simulink model "rct_airframeGS"  (R2016b)
settings: Solver=ode45  StartTime=0.0  StopTime=50  RelTol=1e-3  AbsTol=1e-6
PreLoadFcn:
  | x_ini = 0;
  | h_ini = 10000/3.28084;  % 10,000 ft
  | alpha_ini = 0;
  | theta_ini = 0;
  | v_ini = 700;   % m/s
  | q_ini = 0;
model workspace (MATLAB code in the model file):
  | AirframeData
  | Kp0 = 0.1*ones(11,8);
  | Ki0 = 2*ones(11,8);
  | Ka0 = 0.001*ones(11,8);
  | Kg0 = -1000*ones(11,8);
undefined symbols (not defined in the file or in its folder): Cm_alpha, Cm_el, Cm_q, Cx_alpha, Cz_alpha, Cz_el, d2r, d_ref, fin_max, fin_min, g, S_ref, Thrust
libraries: aerospace x3, simulink x1
settings Model: ExtModeTrigMode=oneshot  ExtModeArmWhenConnect=off  ExtModeAutoUpdateStatusClock=off  Creator=The MathWorks, Inc.  LastModifiedBy=The MathWorks, Inc.
settings DataIOCC: SaveFormat=Array  SignalLoggingName=sigsOut
settings OptimizationCC: BlockReduction=off  BooleanDataType=off  ExpressionDepthLimit=2147483647  InitFltsAndDblsToZero=on  LifeSpan=inf
settings DebuggingCC: SaveWithParameterizedLinksMsg=none  UnderspecifiedInitializationDetection=Classic  MergeDetectMultiDrivingBlocksExec=none  CheckExecutionContextPreStartOutputMsg=on  CheckExecutionContextRuntimeOutputMsg=on  SignalResolutionControl=TryResolveAllWithWarning  MultiTaskDSMMsg=warning  FcnCallInpInsideContextMsg=warning  AllowSymbolicDim=off  StateNameClashWarn=warning  SFUnexpectedBacktrackingDiag=warning  SFNoUnconditionalDefaultTransitionDiag=warning  SFExecutionAtInitializationDiag=none
settings HardwareCC: ProdBitPerPointer=32  ProdBitPerSizeT=32  ProdBitPerPtrDiffT=32  ProdLargestAtomicFloat=None  ProdIntDivRoundTo=Undefined  ProdEndianess=Unspecified  ProdWordSize=32  ProdHWDeviceType=32-bit Generic  TargetUnknown=on
settings ModelReferenceCC: PropagateSignalLabelsOutOfModel=off
settings GRTTargetCC: TargetFcnLib=ansi_tfl_tmw.mat  TargetLangStandard=C89/C90 (ANSI)  GeneratePreprocessorConditionals=Disable all  CombineOutputUpdateFcns=off  GRTInterface=on
settings ConfigComp: CovMetricSettings=dw  CovHtmlReporting=on  CovSaveCumulativeToWorkspaceVar=on  CovSaveSingleToWorkspaceVar=on  CovExternalEMLEnable=off

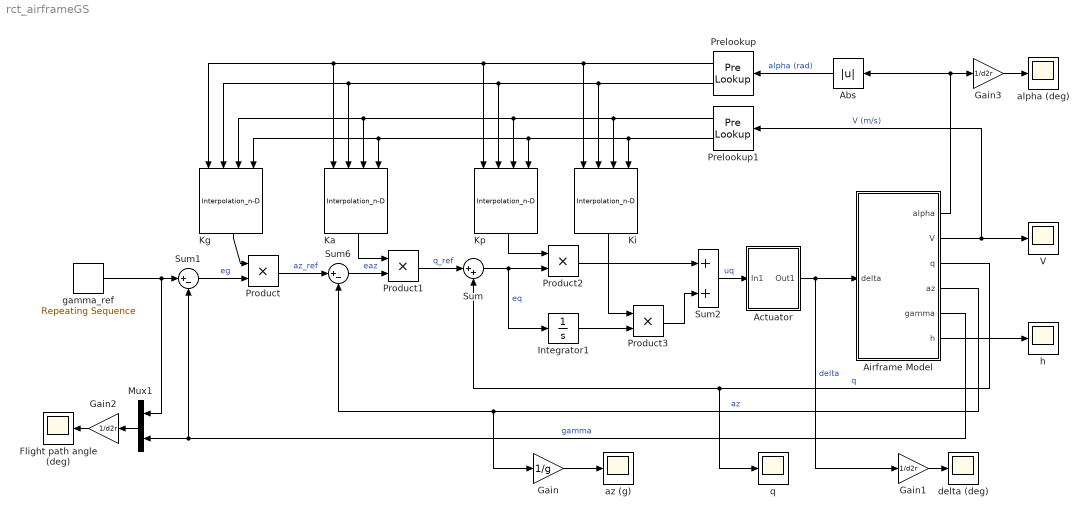
== system rct_airframeGS ==
  Abs : Abs
  Actuator : Subsystem
  Airframe Model : Subsystem
  Flight path angle (deg) : Scope
  Gain : Gain  Gain=1/g
  Gain1 : Gain  Gain=1/d2r
  Gain2 : Gain  Gain=1/d2r
  Gain3 : Gain  Gain=1/d2r
  Integrator1 : Integrator
  Ka : Interpolation_n-D  Table=Ka0  InternalRulePriority=Speed
  Kg : Interpolation_n-D  Table=Kg0  InternalRulePriority=Speed
  Ki : Interpolation_n-D  Table=Ki0  InternalRulePriority=Speed
  Kp : Interpolation_n-D  Table=Kp0  InternalRulePriority=Speed
  Mux1 : Mux  Inputs=2
  Prelookup : PreLookup  BreakpointsData=(0:2:20)*(pi/180)  ExtrapMethod=Linear
  Prelookup1 : PreLookup  BreakpointsData=700:100:1400  ExtrapMethod=Linear
  Product{,1..3} (4 alike) : Product
  Sum : Sum  Inputs=|++  SaturateOnIntegerOverflow=on
  Sum1 : Sum  Inputs=|+-  SaturateOnIntegerOverflow=on
  Sum2 : Sum  SaturateOnIntegerOverflow=on
  Sum6 : Sum  Inputs=|+-  SaturateOnIntegerOverflow=on
  V : Scope
  alpha (deg) : Scope
  az (g) : Scope
  delta (deg) : Scope
  gamma_ref : simulink/Sources/Repeating Sequence  rep_seq_t=[0 6 8 16 20 26 32 40 44 50]  rep_seq_y=[0 0 pi/6 pi/6 -pi/6 -pi/6 pi/4 pi/4 0 0]
  h : Scope
  q : Scope
  wires:
  Sum/1 -> Product2/2, Integrator1/1  "eq"
  Product3/1 -> Sum2/2
  Airframe Model/4(az) -> Gain/1, Sum6/2  "az"
  Airframe Model/1(alpha) -> Abs/1, Gain3/1
  Product2/1 -> Sum2/1
  Product1/1 -> Sum/1  "q_ref"
  Sum6/1 -> Product1/2  "eaz"
  Actuator/1(Out1) -> Airframe Model/1(delta), Gain1/1  "delta"
  Product/1 -> Sum6/1  "az_ref"
  Sum1/1 -> Product/2  "eg"
  Airframe Model/5(gamma) -> Mux1/2, Sum1/2  "gamma"
  Sum2/1 -> Actuator/1(In1)  "uq"
  Airframe Model/3(q) -> q/1, Sum/2  "q"
  gamma_ref/1 -> Sum1/1, Mux1/1
  Gain/1 -> az (g)/1
  Gain1/1 -> delta (deg)/1
  Mux1/1 -> Gain2/1
  Gain2/1 -> Flight path angle (deg)/1
  Gain3/1 -> alpha (deg)/1
  Airframe Model/2(V) -> Prelookup1/1, V/1  "V (m/s)"
  Airframe Model/6(h) -> h/1
  Kg/1 -> Product/1
  Ka/1 -> Product1/1
  Integrator1/1 -> Product3/2
  Kp/1 -> Product2/1
  Ki/1 -> Product3/1
  Abs/1 -> Prelookup/1  "alpha (rad)"
  Prelookup/1 -> Ka/1, Kg/1, Kp/1, Ki/1
  Prelookup/2 -> Ki/2, Kp/2, Ka/2, Kg/2
  Prelookup1/1 -> Kp/3, Kg/3, Ka/3, Ki/3
  Prelookup1/2 -> Ki/4, Kg/4, Ka/4, Kp/4

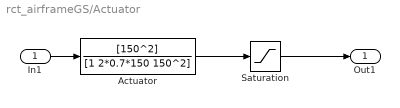
== system rct_airframeGS/Actuator ==
  In1 : Inport
  Actuator : TransferFcn  Numerator=[150^2]  Denominator=[1 2*0.7*150 150^2]
  Saturation : Saturate  UpperLimit=fin_max  LowerLimit=fin_min
  Out1 : Outport
  wires:
  Actuator/1 -> Saturation/1
  In1/1 -> Actuator/1
  Saturation/1 -> Out1/1

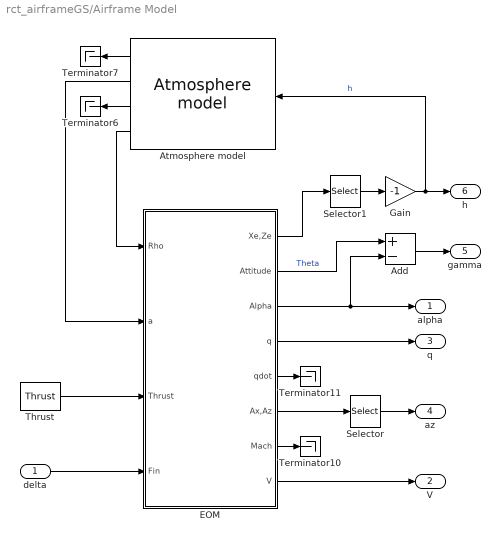
== system rct_airframeGS/Airframe Model ==
  delta : Inport
  Add : Sum  Inputs=+-
  Atmosphere model : aerospace/Atmosphere/Atmosphere model
  EOM : Subsystem
  Gain : Gain  Gain=-1
  Selector : Selector  InputPortWidth=2  IndexOptions=Index vector (dialog)  Indices=[2]  OutputSizes=1
  Selector1 : Selector  InputPortWidth=2  IndexOptions=Index vector (dialog)  Indices=[2]  OutputSizes=1
  Terminator{6..7,10..11} (4 alike) : Terminator
  Thrust : Constant  Value=Thrust
  alpha : Outport  InitialOutput=0
  V : Outport  Port=2  InitialOutput=0
  q : Outport  Port=3  InitialOutput=0
  az : Outport  Port=4  InitialOutput=0
  gamma : Outport  Port=5  InitialOutput=0
  h : Outport  Port=6  InitialOutput=0
  wires:
  Atmosphere model/1 -> Terminator7/1
  Atmosphere model/3 -> Terminator6/1
  delta/1 -> EOM/4(Fin)
  EOM/8(V) -> V/1
  Selector/1 -> az/1
  Atmosphere model/2 -> EOM/2(a)
  Atmosphere model/4 -> EOM/1(Rho)
  EOM/7(Mach) -> Terminator10/1
  EOM/5(qdot) -> Terminator11/1
  EOM/4(q) -> q/1
  Thrust/1 -> EOM/3(Thrust)
  EOM/3(Alpha) -> alpha/1, Add/2
  EOM/6(Ax,Az) -> Selector/1
  EOM/2(Attitude) -> Add/1  "Theta"
  Add/1 -> gamma/1
  EOM/1(Xe,Ze) -> Selector1/1
  Selector1/1 -> Gain/1
  Gain/1 -> Atmosphere model/1, h/1  "h"

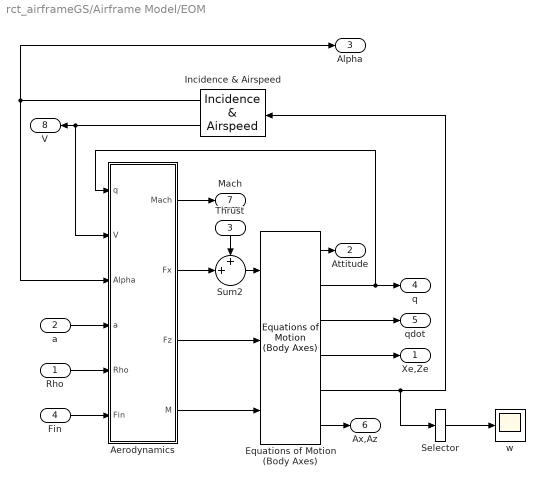
== system rct_airframeGS/Airframe Model/EOM ==
  Rho : Inport
  a : Inport  Port=2
  Thrust : Inport  Port=3
  Fin : Inport  Port=4
  " Equations of Motion (Body Axes)" : aerospace/3DoF Equations of Motion / Equations of Motion (Body Axes)  v_ini=v_ini  theta_ini=theta_ini  alpha_ini=alpha_ini  q_ini=q_ini  pos_ini=[x_ini -h_ini]  mass=mass  Iyy=Iyy  g=g
  Aerodynamics : Subsystem
  Incidence & Airspeed : aerospace/3DoF Equations of Motion /Incidence  & Airspeed
  Selector : Selector  InputPortWidth=2  IndexOptions=Index vector (dialog)  Indices=[2]  OutputSizes=1
  Sum2 : Sum  Inputs=++|  SaturateOnIntegerOverflow=on  InputSameDT=on  OutDataTypeStr=Inherit: Same as first input
  w : Scope
  Xe,Ze : Outport  InitialOutput=0
  Attitude : Outport  Port=2  InitialOutput=0
  Alpha : Outport  Port=3  InitialOutput=0
  q : Outport  Port=4  InitialOutput=0
  qdot : Outport  Port=5  InitialOutput=0
  Ax,Az : Outport  Port=6  InitialOutput=0
  Mach : Outport  Port=7  InitialOutput=0
  V : Outport  Port=8  InitialOutput=0
  wires:
  " Equations of Motion (Body Axes)"/5 -> Selector/1, Incidence & Airspeed/1
  " Equations of Motion (Body Axes)"/6 -> Ax,Az/1
  " Equations of Motion (Body Axes)"/4 -> Xe,Ze/1
  " Equations of Motion (Body Axes)"/1 -> Attitude/1
  " Equations of Motion (Body Axes)"/3 -> qdot/1
  " Equations of Motion (Body Axes)"/2 -> Aerodynamics/1(q), q/1
  Thrust/1 -> Sum2/1
  Aerodynamics/2(Fx) -> Sum2/2
  Aerodynamics/3(Fz) -> " Equations of Motion (Body Axes)"/2
  Incidence & Airspeed/2 -> Aerodynamics/2(V), V/1
  Fin/1 -> Aerodynamics/6(Fin)
  a/1 -> Aerodynamics/4(a)
  Rho/1 -> Aerodynamics/5(Rho)
  Incidence & Airspeed/1 -> Alpha/1, Aerodynamics/3(Alpha)
  Sum2/1 -> " Equations of Motion (Body Axes)"/1
  Aerodynamics/4(" M") -> " Equations of Motion (Body Axes)"/3
  Aerodynamics/1(" Mach") -> Mach/1
  Selector/1 -> w/1

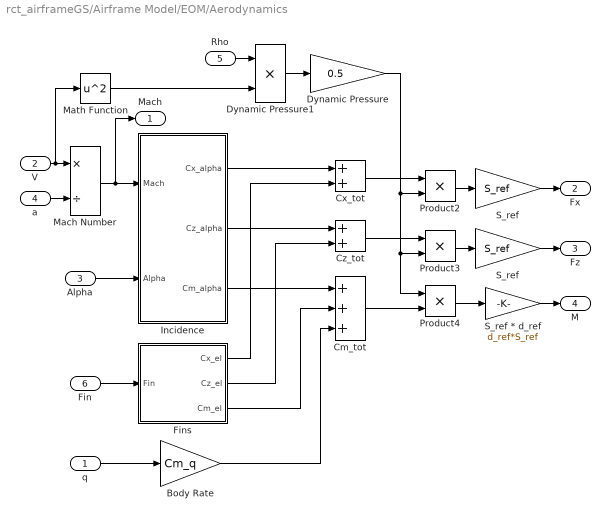
== system rct_airframeGS/Airframe Model/EOM/Aerodynamics ==
  q : Inport
  V : Inport  Port=2
  Alpha : Inport  Port=3
  a : Inport  Port=4
  Rho : Inport  Port=5
  Fin : Inport  Port=6
  Body Rate : Gain  Gain=Cm_q  SaturateOnIntegerOverflow=on  OutDataTypeStr=Inherit: Same as input  ParamDataTypeStr=Inherit: Same as input
  Cm_tot : Sum  Inputs=+++  SaturateOnIntegerOverflow=on  InputSameDT=on  OutDataTypeStr=Inherit: Same as first input
  Cx_tot : Sum  SaturateOnIntegerOverflow=on  InputSameDT=on  OutDataTypeStr=Inherit: Same as first input
  Cz_tot : Sum  SaturateOnIntegerOverflow=on  InputSameDT=on  OutDataTypeStr=Inherit: Same as first input
  Dynamic Pressure : Gain  Gain=0.5  SaturateOnIntegerOverflow=on  OutDataTypeStr=Inherit: Same as input  ParamDataTypeStr=Inherit: Same as input
  Dynamic Pressure1 : Product  SaturateOnIntegerOverflow=on  InputSameDT=on  OutDataTypeStr=Inherit: Same as first input
  Fins : Subsystem
  Incidence : Subsystem
  Mach Number : Product  Inputs=*/  SaturateOnIntegerOverflow=on  InputSameDT=on  OutDataTypeStr=Inherit: Same as first input
  Math Function : Math  Operator=square  SaturateOnIntegerOverflow=on
  Product2 : Product  SaturateOnIntegerOverflow=on  InputSameDT=on  OutDataTypeStr=Inherit: Same as first input
  Product3 : Product  SaturateOnIntegerOverflow=on  InputSameDT=on  OutDataTypeStr=Inherit: Same as first input
  Product4 : Product  SaturateOnIntegerOverflow=on  InputSameDT=on  OutDataTypeStr=Inherit: Same as first input
  S_ref : Gain  Gain=S_ref  SaturateOnIntegerOverflow=on  OutDataTypeStr=Inherit: Same as input  ParamDataTypeStr=Inherit: Same as input
  S_ref * d_ref : Gain  Gain=d_ref*S_ref  SaturateOnIntegerOverflow=on  OutDataTypeStr=Inherit: Same as input  ParamDataTypeStr=Inherit: Same as input
  "S_ref " : Gain  Gain=S_ref  SaturateOnIntegerOverflow=on  OutDataTypeStr=Inherit: Same as input  ParamDataTypeStr=Inherit: Same as input
  " Mach" : Outport  InitialOutput=0
  Fx : Outport  Port=2  InitialOutput=[0]
  Fz : Outport  Port=3  InitialOutput=0
  " M" : Outport  Port=4  InitialOutput=0
  wires:
  Mach Number/1 -> Incidence/1(Mach), " Mach"/1
  q/1 -> Body Rate/1
  Cm_tot/1 -> Product4/2
  Product4/1 -> S_ref * d_ref/1
  S_ref * d_ref/1 -> " M"/1
  Fin/1 -> Fins/1(Fin)
  "S_ref "/1 -> Fz/1
  Product3/1 -> "S_ref "/1
  S_ref/1 -> Fx/1
  Product2/1 -> S_ref/1
  Cz_tot/1 -> Product3/1
  Cx_tot/1 -> Product2/1
  Alpha/1 -> Incidence/2(Alpha)
  a/1 -> Mach Number/2
  Body Rate/1 -> Cm_tot/3
  Fins/3(Cm_el) -> Cm_tot/2
  Incidence/3(Cm_alpha) -> Cm_tot/1
  Fins/2(Cz_el) -> Cz_tot/2
  Incidence/2(Cz_alpha) -> Cz_tot/1
  Fins/1(Cx_el) -> Cx_tot/2
  Incidence/1(Cx_alpha) -> Cx_tot/1
  V/1 -> Mach Number/1, Math Function/1
  Dynamic Pressure/1 -> Product4/1, Product3/2, Product2/2
  Dynamic Pressure1/1 -> Dynamic Pressure/1
  Rho/1 -> Dynamic Pressure1/1
  Math Function/1 -> Dynamic Pressure1/2

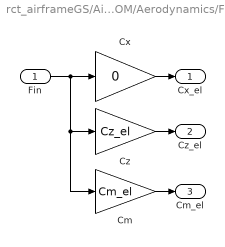
== system rct_airframeGS/Airframe Model/EOM/Aerodynamics/Fins ==
  Fin : Inport
  Cm : Gain  Gain=Cm_el  SaturateOnIntegerOverflow=on  OutDataTypeStr=Inherit: Same as input  ParamDataTypeStr=Inherit: Same as input
  Cx : Gain  Gain=0  SaturateOnIntegerOverflow=on  OutDataTypeStr=Inherit: Same as input  ParamDataTypeStr=Inherit: Same as input
  Cz : Gain  Gain=Cz_el  SaturateOnIntegerOverflow=on  OutDataTypeStr=Inherit: Same as input  ParamDataTypeStr=Inherit: Same as input
  Cx_el : Outport  InitialOutput=0
  Cz_el : Outport  Port=2  InitialOutput=0
  Cm_el : Outport  Port=3  InitialOutput=0
  wires:
  Cz/1 -> Cz_el/1
  Cm/1 -> Cm_el/1
  Cx/1 -> Cx_el/1
  Fin/1 -> Cz/1, Cm/1, Cx/1

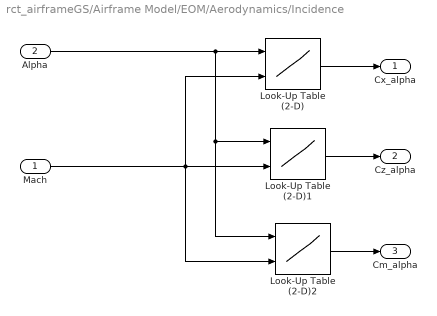
== system rct_airframeGS/Airframe Model/EOM/Aerodynamics/Incidence ==
  Mach : Inport
  Alpha : Inport  Port=2
  Look-Up Table (2-D) : Lookup2D  RowIndex=alpha_vec  ColumnIndex=Mach_vec  Table=Cx_alpha  SaturateOnIntegerOverflow=on
  Look-Up Table (2-D)1 : Lookup2D  RowIndex=alpha_vec  ColumnIndex=Mach_vec  Table=Cz_alpha  SaturateOnIntegerOverflow=on
  Look-Up Table (2-D)2 : Lookup2D  RowIndex=alpha_vec  ColumnIndex=Mach_vec  Table=Cm_alpha  SaturateOnIntegerOverflow=on
  Cx_alpha : Outport  InitialOutput=0
  Cz_alpha : Outport  Port=2  InitialOutput=0
  Cm_alpha : Outport  Port=3  InitialOutput=0
  wires:
  Mach/1 -> Look-Up Table (2-D)2/2, Look-Up Table (2-D)1/2, Look-Up Table (2-D)/2
  Alpha/1 -> Look-Up Table (2-D)2/1, Look-Up Table (2-D)1/1, Look-Up Table (2-D)/1
  Look-Up Table (2-D)2/1 -> Cm_alpha/1
  Look-Up Table (2-D)1/1 -> Cz_alpha/1
  Look-Up Table (2-D)/1 -> Cx_alpha/1
